simulink model "Water_tank_simulink"  (R2019b)
settings: Solver=VariableStepAuto  StartTime=0.0  StopTime=800  RelTol=1e-3
settings Model: Creator=Δημήτρης  LastModifiedBy=Δημήτρης

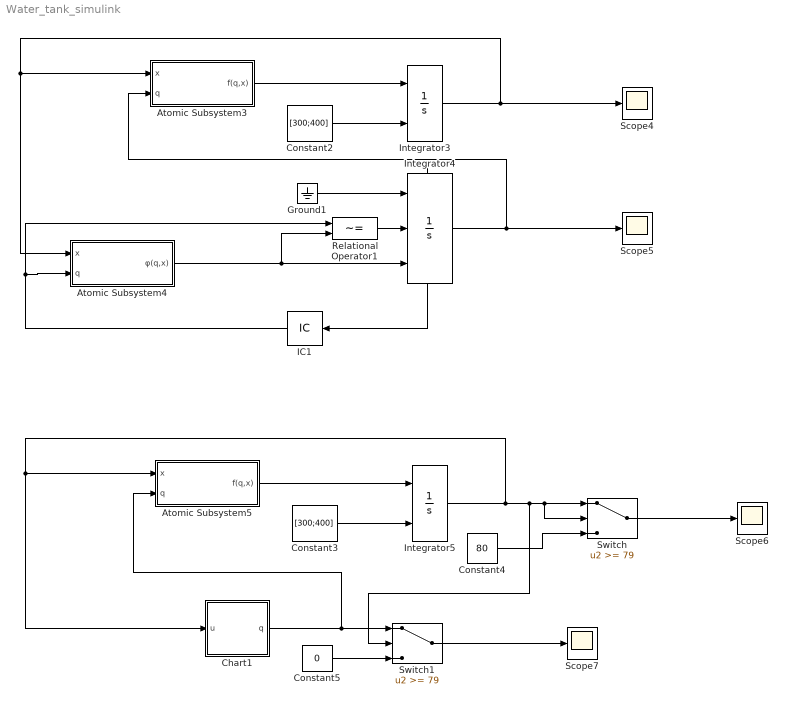
== system Water_tank_simulink ==
  Atomic Subsystem3 : Subsystem  TreatAsAtomicUnit=on
  Atomic Subsystem4 : Subsystem  TreatAsAtomicUnit=on
  Atomic Subsystem5 : Subsystem  TreatAsAtomicUnit=on
  Chart1 : Stateflow chart  BlockKeywords=__PRM__SERIALIZED__DATA__:Stateflow Chart,Stateflow Diagram  TreatAsAtomicUnit=on
  Constant2 : Constant  Value=[300;400]
  Constant3 : Constant  Value=[300;400]
  Constant4 : Constant  Value=80
  Constant5 : Constant  Value=0
  Ground1 : Ground
  IC1 : InitialCondition
  Integrator3 : Integrator  InitialConditionSource=external
  Integrator4 : Integrator  ExternalReset=rising  InitialConditionSource=external  ShowStatePort=on
  Integrator5 : Integrator  InitialConditionSource=external
  Relational Operator1 : RelationalOperator  Operator=~=  OutDataTypeStr=boolean  RndMeth=Simplest
  Scope{4..7} (4 alike) : Scope
  Switch : Switch  Threshold=79  InputSameDT=on
  Switch1 : Switch  Threshold=79  InputSameDT=on
  wires:
  Relational Operator1/1 -> Integrator4/2
  Atomic Subsystem4/1(φ(q,x)) -> Integrator4/3, Relational Operator1/2
  Ground1/1 -> Integrator4/1
  Atomic Subsystem5/1("f(q,x) ") -> Integrator5/1
  Integrator5/1 -> Switch1/2, Switch/2, Switch/1, Chart1/1(u), Atomic Subsystem5/1(x)
  Constant3/1 -> Integrator5/2
  Integrator3/1 -> Scope4/1, Atomic Subsystem4/1(x), Atomic Subsystem3/1(x)
  Integrator4/1 -> Scope5/1, Atomic Subsystem3/2(q)
  Constant2/1 -> Integrator3/2
  Atomic Subsystem3/1("f(q,x) ") -> Integrator3/1
  IC1/1 -> Atomic Subsystem4/2(q), Relational Operator1/1
  Integrator4/State -> IC1/1
  Chart1/1(q) -> Atomic Subsystem5/2(q), Switch1/1
  Switch1/1 -> Scope7/1
  Constant5/1 -> Switch1/3
  Constant4/1 -> Switch/3
  Switch/1 -> Scope6/1

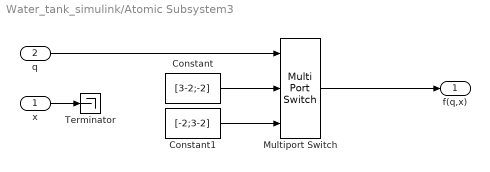
== system Water_tank_simulink/Atomic Subsystem3 ==
  x : Inport
  q : Inport  Port=2
  Constant : Constant  Value=[3-2;-2]
  Constant1 : Constant  Value=[-2;3-2]
  Multiport Switch : MultiPortSwitch  Inputs=2  DiagnosticForDefault=None
  Terminator : Terminator
  "f(q,x) " : Outport
  wires:
  Multiport Switch/1 -> "f(q,x) "/1
  x/1 -> Terminator/1
  q/1 -> Multiport Switch/1
  Constant1/1 -> Multiport Switch/3
  Constant/1 -> Multiport Switch/2

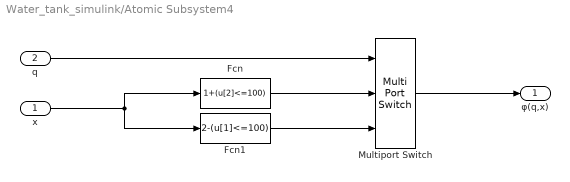
== system Water_tank_simulink/Atomic Subsystem4 ==
  x : Inport
  q : Inport  Port=2
  Fcn : Fcn  Expr=1+(u[2]<=100)
  Fcn1 : Fcn  Expr=2-(u[1]<=100)
  Multiport Switch : MultiPortSwitch  Inputs=2  DiagnosticForDefault=None
  φ(q,x) : Outport
  wires:
  q/1 -> Multiport Switch/1
  x/1 -> Fcn/1, Fcn1/1
  Fcn/1 -> Multiport Switch/2
  Fcn1/1 -> Multiport Switch/3
  Multiport Switch/1 -> φ(q,x)/1

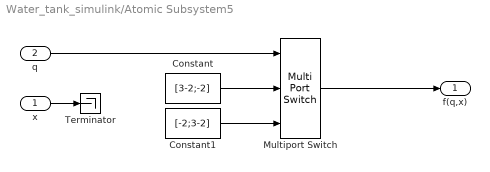
== system Water_tank_simulink/Atomic Subsystem5 ==
  x : Inport
  q : Inport  Port=2
  Constant : Constant  Value=[3-2;-2]
  Constant1 : Constant  Value=[-2;3-2]
  Multiport Switch : MultiPortSwitch  Inputs=2  DiagnosticForDefault=None
  Terminator : Terminator
  "f(q,x) " : Outport
  wires:
  Constant/1 -> Multiport Switch/2
  Constant1/1 -> Multiport Switch/3
  q/1 -> Multiport Switch/1
  x/1 -> Terminator/1
  Multiport Switch/1 -> "f(q,x) "/1

== stateflow chart Water_tank_simulink/Chart1 ==
  state on
    entry:q=1;
  state off
    entry:q=0;
  (default) -> on
  on -> off : [u(2)<=80]
  off -> on : [u(1)<=80]
  data: u input; q output
